simulink model "slave_exec"  (Simulink 3.00)
libraries: execlib x6

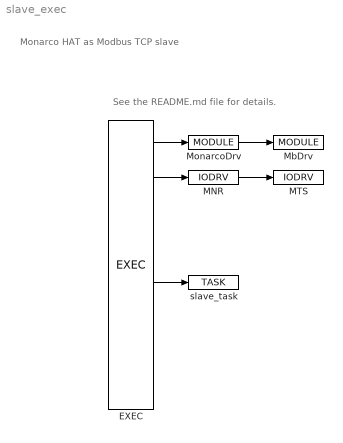
== system slave_exec ==
  note: See the README.md file for details.
  note: Monarco HAT as Modbus TCP
      | slave
  EXEC : execlib/EXEC  target=Generic target device  tick=0.005  ntick0=2  ntick1=50  ntick2=100  ntick3=1200  pri0=5  pri1=9  pri2=13  pri3=18
  MNR : execlib/IODRV  module=MonarcoDrv  classname=MonarcoHatDrv  cfgname=monarco_cfg.rio  factor=2  stack=10240  pri=3  timer=off
  MTS : execlib/IODRV  module=MbDrv  classname=MtsDrv  cfgname=mbtcp_slave_cfg.rio  factor=2  stack=10240  pri=3  timer=off
  MbDrv : execlib/MODULE
  MonarcoDrv : execlib/MODULE
  slave_task : execlib/TASK  factor=1  start=1  stop=2  stack=10240  MDLOPEN=on
  wires:
  EXEC/1 -> MonarcoDrv/1
  EXEC/2 -> MNR/1
  EXEC/5 -> slave_task/1
  MNR/1 -> MTS/1
  MonarcoDrv/1 -> MbDrv/1
